simulink model "serialControl"  (R2024a)
settings: Solver=ode5  StartTime=0.0  StopTime=inf  FixedStep=1e-3
model workspace (MAT data in the model file):
  I_idq_regulator = 1
  Id_setpoint = 1
  Iq_setpoint = 1
  OL_Freq_Command = 1
  P_idq_regulator = 1
libraries: instrumentseriallib x7, svdutilitieslib x6, simulink x5
settings Model: PauseTimes=3  Creator=lrada  LastModifiedBy=lrada
settings HardwareCC: ProdBitPerLong=64  ProdHWDeviceType=Intel->x86-64 (Linux 64)
settings RTWCC: Description=Simulink Desktop Real-Time  SystemTargetFile=sldrt.tlc  TemplateMakefile=sldrt.tmf  RTWCompilerOptimization=on
settings CodeAppCC: MaxIdLength=95
settings SimulinkDesktopRealTimeCC: TargetLibSuffix=_sldrt.a  TargetPreCompLibLocation=C:\Program Files\MATLAB\R2024a\toolbox\sldrt\lib\win64

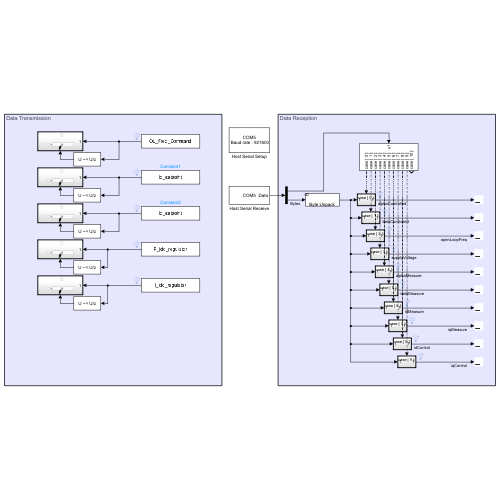
[thumbnail: Simulink's stored preview of the top-level diagram]
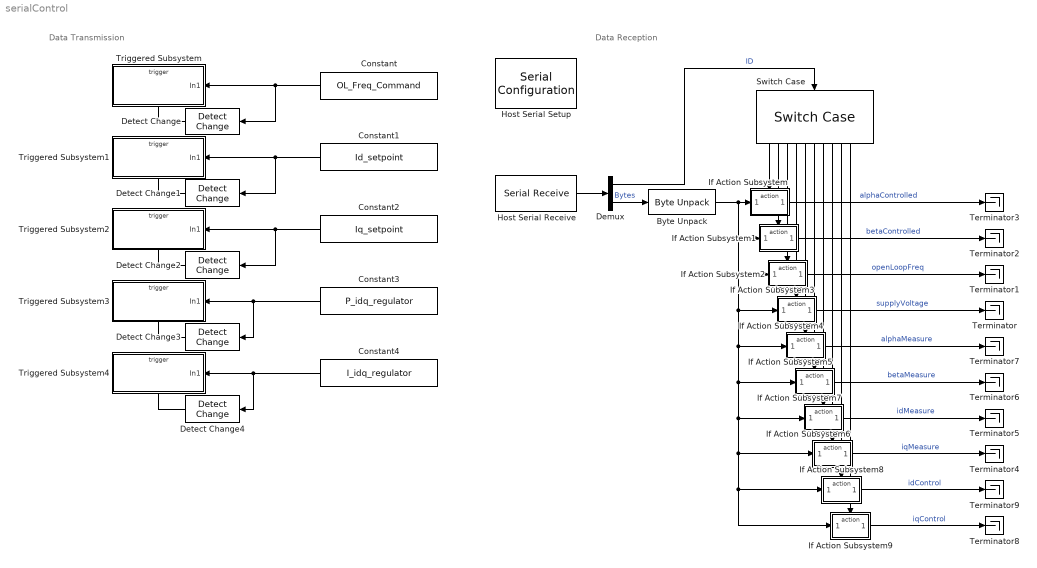
== system serialControl ==
  note: Data Reception
  note: Data Transmission
  Byte Unpack : svdutilitieslib/Byte Unpack  dimensions={[1]}  datatypes={'single'}  byteAlign=1  blockPlatform=arduinoert
      settings: LibrarySourceBlock=mcblib/Signal Management/Byte Unpack
  Constant : Constant  Value=OL_Freq_Command  OutDataTypeStr=single
  Constant1 : Constant  Value=Id_setpoint  OutDataTypeStr=single
  Constant2 : Constant  Value=Iq_setpoint  OutDataTypeStr=single
  Constant3 : Constant  Value=P_idq_regulator  OutDataTypeStr=single
  Constant4 : Constant  Value=I_idq_regulator  OutDataTypeStr=single
  Demux : Demux  Outputs=[1 4]
  Detect Change{,1..4} (5 alike) : simulink/Logic and Bit Operations/Detect Change  vinit=0  OutDataTypeStr=boolean
  Host Serial Receive : instrumentseriallib/Serial Receive  PortSel=COM5  Port=COM5  ComPort=COM5  DataType=uint8  SaveDataType=uint8  ToggleHeader=off  Header='S'  ToggleDataSize=on  DataSize=5  ToggleTerminator=on  Terminator=Custom terminator  CustomTerminator='EOF'  InputFormat=Column major  EnableBlockingMode=on  ActionDataUnavailable=Output last received value  ActionWhenDataUnavailable=Output last received value  CustomValue=0  SampleTime=1e-3  SimulateUsing=Interpreted execution  BlockInModel=on  aMode=5
      settings: LibrarySourceBlock=mcblib/Protection and Diagnostics/Host Serial Receive
  Host Serial Setup : instrumentseriallib/Serial Configuration  Priority=-99  PortSel=COM5  Port=COM5  ComPort=COM5  BaudRate=921600  DataBits=8  Parity=none  StopBits=1  ByteOrder=little-endian  FlowControl=none  Timeout=1.0  SimulateUsing=Interpreted execution  BlockInModel=on  aMode=5
      settings: LibrarySourceBlock=mcblib/Protection and Diagnostics/Host Serial Setup
  If Action Subsystem : Subsystem  TreatAsAtomicUnit=on
  If Action Subsystem1 : Subsystem  TreatAsAtomicUnit=on
  If Action Subsystem2 : Subsystem  TreatAsAtomicUnit=on
  If Action Subsystem3 : Subsystem  TreatAsAtomicUnit=on
  If Action Subsystem4 : Subsystem  TreatAsAtomicUnit=on
  If Action Subsystem5 : Subsystem  TreatAsAtomicUnit=on
  If Action Subsystem6 : Subsystem  TreatAsAtomicUnit=on
  If Action Subsystem7 : Subsystem  TreatAsAtomicUnit=on
  If Action Subsystem8 : Subsystem  TreatAsAtomicUnit=on
  If Action Subsystem9 : Subsystem  TreatAsAtomicUnit=on
  Switch Case : SwitchCase  CaseConditions={0,1,2,3,4,5,6,7,8,9,10}  ShowDefaultCase=off
  Terminator{,1..9} (10 alike) : Terminator
  Triggered Subsystem : Subsystem  TreatAsAtomicUnit=on
  Triggered Subsystem1 : Subsystem  TreatAsAtomicUnit=on
  Triggered Subsystem2 : Subsystem  TreatAsAtomicUnit=on
  Triggered Subsystem3 : Subsystem  TreatAsAtomicUnit=on
  Triggered Subsystem4 : Subsystem  TreatAsAtomicUnit=on
  wires:
  Demux/1 -> Switch Case/1  "ID"
  Demux/2 -> Byte Unpack/1  "Bytes"
  Switch Case/1 -> If Action Subsystem/Action
  Switch Case/2 -> If Action Subsystem1/Action
  Switch Case/3 -> If Action Subsystem2/Action
  Switch Case/4 -> If Action Subsystem3/Action
  Host Serial Receive/1 -> Demux/1
  If Action Subsystem3/1(Out1) -> Terminator/1  "supplyVoltage"
  If Action Subsystem2/1(Out1) -> Terminator1/1  "openLoopFreq"
  If Action Subsystem1/1(Out1) -> Terminator2/1  "betaControlled"
  If Action Subsystem/1(Out1) -> Terminator3/1  "alphaControlled"
  Constant/1 -> Detect Change/1, Triggered Subsystem/1(In1)
  Detect Change/1 -> Triggered Subsystem/Trigger
  If Action Subsystem4/1(Out1) -> Terminator7/1  "alphaMeasure"
  Switch Case/6 -> If Action Subsystem5/Action
  If Action Subsystem6/1(Out1) -> Terminator4/1  "iqMeasure"
  If Action Subsystem5/1(Out1) -> Terminator6/1  "betaMeasure"
  Switch Case/5 -> If Action Subsystem4/Action
  Switch Case/7 -> If Action Subsystem7/Action
  Switch Case/8 -> If Action Subsystem6/Action
  If Action Subsystem7/1(Out1) -> Terminator5/1  "idMeasure"
  Switch Case/9 -> If Action Subsystem8/Action
  Byte Unpack/1 -> If Action Subsystem/1(In1), If Action Subsystem1/1(In1), If Action Subsystem2/1(In1), If Action Subsystem3/1(In1), If Action Subsystem4/1(In1), If Action Subsystem5/1(In1), If Action Subsystem7/1(In1), If Action Subsystem9/1(In1), If Action Subsystem8/1(In1), If Action Subsystem6/1(In1)
  Switch Case/10 -> If Action Subsystem9/Action
  If Action Subsystem9/1(Out1) -> Terminator8/1  "iqControl"
  If Action Subsystem8/1(Out1) -> Terminator9/1  "idControl"
  Detect Change1/1 -> Triggered Subsystem1/Trigger
  Constant1/1 -> Detect Change1/1, Triggered Subsystem1/1(In1)
  Constant2/1 -> Detect Change2/1, Triggered Subsystem2/1(In1)
  Detect Change2/1 -> Triggered Subsystem2/Trigger
  Detect Change3/1 -> Triggered Subsystem3/Trigger
  Constant3/1 -> Detect Change3/1, Triggered Subsystem3/1(In1)
  Constant4/1 -> Detect Change4/1, Triggered Subsystem4/1(In1)
  Detect Change4/1 -> Triggered Subsystem4/Trigger

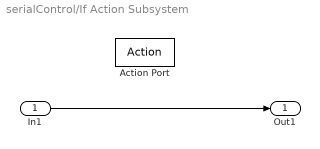
== system serialControl/If Action Subsystem ==
  In1 : Inport
  Action Port : ActionPort  ActionPortLabel=case [ 0 ]:
  Out1 : Outport
  wires:
  In1/1 -> Out1/1

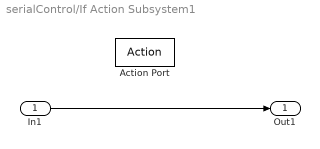
== system serialControl/If Action Subsystem1 ==
  In1 : Inport
  Action Port : ActionPort  ActionPortLabel=case [ 1 ]:
  Out1 : Outport
  wires:
  In1/1 -> Out1/1

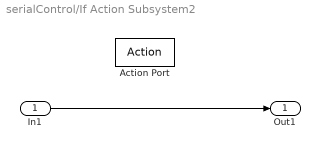
== system serialControl/If Action Subsystem2 ==
  In1 : Inport
  Action Port : ActionPort  ActionPortLabel=case [ 2 ]:
  Out1 : Outport
  wires:
  In1/1 -> Out1/1

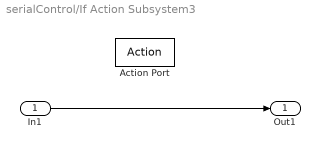
== system serialControl/If Action Subsystem3 ==
  In1 : Inport
  Action Port : ActionPort  ActionPortLabel=case [ 3 ]:
  Out1 : Outport
  wires:
  In1/1 -> Out1/1

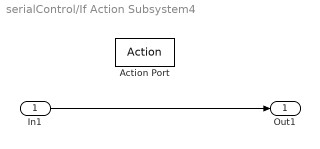
== system serialControl/If Action Subsystem4 ==
  In1 : Inport
  Action Port : ActionPort  ActionPortLabel=case [ 4 ]:
  Out1 : Outport
  wires:
  In1/1 -> Out1/1

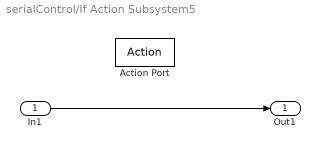
== system serialControl/If Action Subsystem5 ==
  In1 : Inport
  Action Port : ActionPort  ActionPortLabel=case [ 5 ]:
  Out1 : Outport
  wires:
  In1/1 -> Out1/1

== system serialControl/If Action Subsystem6 ==
  In1 : Inport
  Action Port : ActionPort  ActionPortLabel=case [ 7 ]:
  Out1 : Outport
  wires:
  In1/1 -> Out1/1

== system serialControl/If Action Subsystem7 ==
  In1 : Inport
  Action Port : ActionPort  ActionPortLabel=case [ 6 ]:
  Out1 : Outport
  wires:
  In1/1 -> Out1/1

== system serialControl/If Action Subsystem8 ==
  In1 : Inport
  Action Port : ActionPort  ActionPortLabel=case [ 8 ]:
  Out1 : Outport
  wires:
  In1/1 -> Out1/1

== system serialControl/If Action Subsystem9 ==
  In1 : Inport
  Action Port : ActionPort  ActionPortLabel=case [ 9 ]:
  Out1 : Outport
  wires:
  In1/1 -> Out1/1

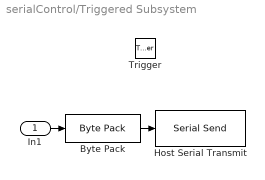
== system serialControl/Triggered Subsystem ==
  In1 : Inport
  Trigger : TriggerPort  VariantControl=(inherit)
  Byte Pack : svdutilitieslib/Byte Pack  maskPackedDataType=uint8  datatypes={'single'}  byteAlign=4  blockPlatform=arduinoert
      settings: LibrarySourceBlock=mcblib/Signal Management/Byte Pack
  Host Serial Transmit : instrumentseriallib/Serial Send  PortSel=COM5  Port=COM5  ComPort=COM5  Header=0  Terminator=<none>  CustomTerminator='E'  EnableBlockingMode=on  SimulateUsing=Interpreted execution  BlockInModel=on  aMode=5
      settings: LibrarySourceBlock=mcblib/Protection and Diagnostics/Host Serial Transmit
  wires:
  Byte Pack/1 -> Host Serial Transmit/1
  In1/1 -> Byte Pack/1

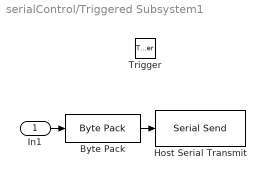
== system serialControl/Triggered Subsystem1 ==
  In1 : Inport
  Trigger : TriggerPort  VariantControl=(inherit)
  Byte Pack : svdutilitieslib/Byte Pack  maskPackedDataType=uint8  datatypes={'single'}  byteAlign=4  blockPlatform=arduinoert
      settings: LibrarySourceBlock=mcblib/Signal Management/Byte Pack
  Host Serial Transmit : instrumentseriallib/Serial Send  PortSel=COM5  Port=COM5  ComPort=COM5  Header=1  Terminator=<none>  CustomTerminator='E'  EnableBlockingMode=on  SimulateUsing=Interpreted execution  BlockInModel=on  aMode=5
      settings: LibrarySourceBlock=mcblib/Protection and Diagnostics/Host Serial Transmit
  wires:
  Byte Pack/1 -> Host Serial Transmit/1
  In1/1 -> Byte Pack/1

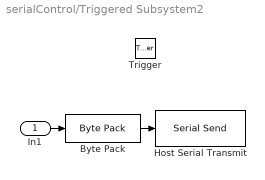
== system serialControl/Triggered Subsystem2 ==
  In1 : Inport
  Trigger : TriggerPort  VariantControl=(inherit)
  Byte Pack : svdutilitieslib/Byte Pack  maskPackedDataType=uint8  datatypes={'single'}  byteAlign=4  blockPlatform=arduinoert
      settings: LibrarySourceBlock=mcblib/Signal Management/Byte Pack
  Host Serial Transmit : instrumentseriallib/Serial Send  PortSel=COM5  Port=COM5  ComPort=COM5  Header=2  Terminator=<none>  CustomTerminator='E'  EnableBlockingMode=on  SimulateUsing=Interpreted execution  BlockInModel=on  aMode=5
      settings: LibrarySourceBlock=mcblib/Protection and Diagnostics/Host Serial Transmit
  wires:
  Byte Pack/1 -> Host Serial Transmit/1
  In1/1 -> Byte Pack/1

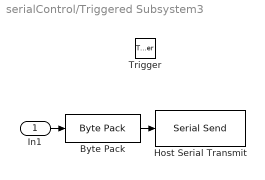
== system serialControl/Triggered Subsystem3 ==
  In1 : Inport
  Trigger : TriggerPort  VariantControl=(inherit)
  Byte Pack : svdutilitieslib/Byte Pack  maskPackedDataType=uint8  datatypes={'single'}  byteAlign=4  blockPlatform=arduinoert
      settings: LibrarySourceBlock=mcblib/Signal Management/Byte Pack
  Host Serial Transmit : instrumentseriallib/Serial Send  PortSel=COM5  Port=COM5  ComPort=COM5  Header=3  Terminator=<none>  CustomTerminator='E'  EnableBlockingMode=on  SimulateUsing=Interpreted execution  BlockInModel=on  aMode=5
      settings: LibrarySourceBlock=mcblib/Protection and Diagnostics/Host Serial Transmit
  wires:
  Byte Pack/1 -> Host Serial Transmit/1
  In1/1 -> Byte Pack/1

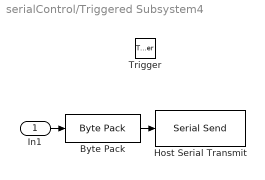
== system serialControl/Triggered Subsystem4 ==
  In1 : Inport
  Trigger : TriggerPort  VariantControl=(inherit)
  Byte Pack : svdutilitieslib/Byte Pack  maskPackedDataType=uint8  datatypes={'single'}  byteAlign=4  blockPlatform=arduinoert
      settings: LibrarySourceBlock=mcblib/Signal Management/Byte Pack
  Host Serial Transmit : instrumentseriallib/Serial Send  PortSel=COM5  Port=COM5  ComPort=COM5  Header=4  Terminator=<none>  CustomTerminator='E'  EnableBlockingMode=on  SimulateUsing=Interpreted execution  BlockInModel=on  aMode=5
      settings: LibrarySourceBlock=mcblib/Protection and Diagnostics/Host Serial Transmit
  wires:
  Byte Pack/1 -> Host Serial Transmit/1
  In1/1 -> Byte Pack/1
